simulink model "Experiment1_model"  (R2022a)
settings: Solver=FixedStepAuto  StartTime=0.0  StopTime=20  RelTol=1e-3
libraries: slpidlib x32, slctrlblks x18
(part 1 of 5)
settings Model: Creator=luca9  LastModifiedBy=luca9

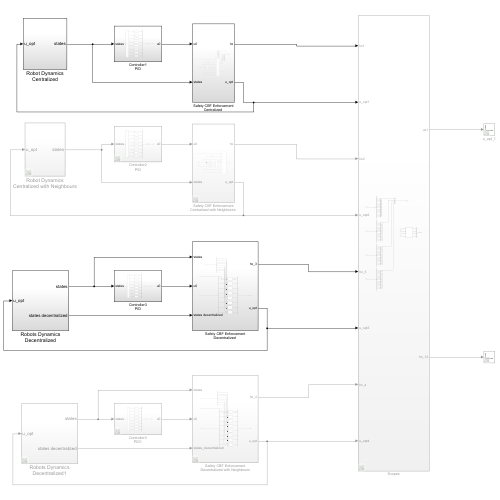
[thumbnail: Simulink's stored preview of the top-level diagram]
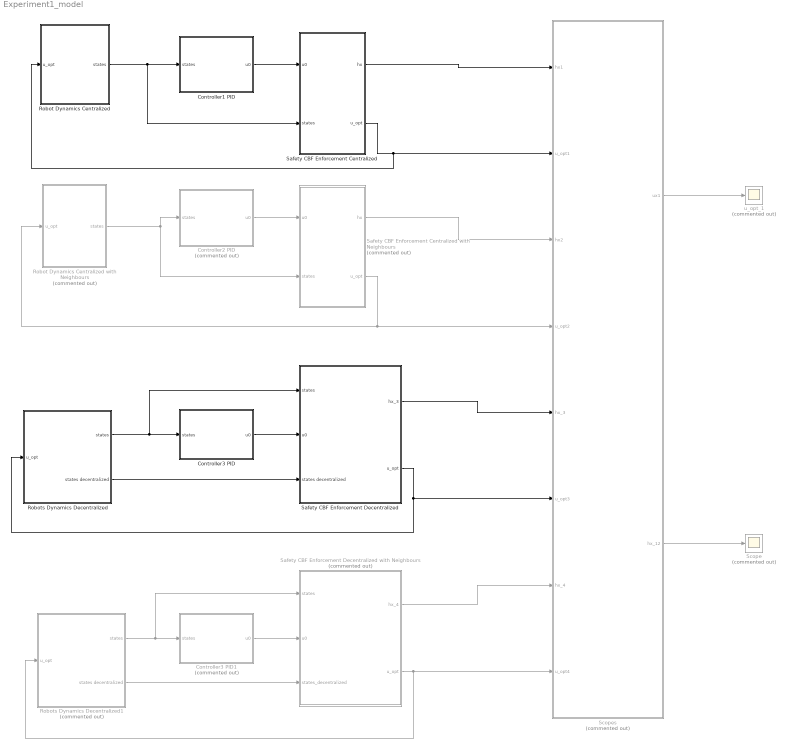
== system Experiment1_model ==
  Controller1 PID : Subsystem
  Controller2 PID : Subsystem  Commented=on
  Controller3 PID : Subsystem
  Controller3 PID1 : Subsystem  Commented=on
  "Robot Dynamics Centralized " : Subsystem
  Robot Dynamics Centralized with Neighbours : Subsystem  Commented=on
  Robots Dynamics Decentralized : Subsystem
  Robots Dynamics Decentralized1 : Subsystem  Commented=on
  "Safety CBF Enforcement Centralized " : Subsystem
  "Safety CBF Enforcement Centralized with Neighbours " : Subsystem  Commented=on
  "Safety CBF Enforcement Decentralized " : Subsystem
  "Safety CBF Enforcement Decentralized with Neighbours " : Subsystem  Commented=on
  Scope : Scope  Commented=on
  Scopes : Subsystem  Commented=on
  u_opt_1 : Scope  Commented=on
  wires:
  Controller1 PID/1(u0) -> "Safety CBF Enforcement Centralized "/1(u0)
  "Robot Dynamics Centralized "/1(states) -> Controller1 PID/1(states), "Safety CBF Enforcement Centralized "/2(states)
  Robots Dynamics Decentralized/1(states) -> "Safety CBF Enforcement Decentralized "/1(states), Controller3 PID/1(states)
  "Safety CBF Enforcement Centralized "/2(u_opt) -> "Robot Dynamics Centralized "/1(u_opt), Scopes/2(u_opt1)
  "Safety CBF Enforcement Centralized with Neighbours "/2(u_opt) -> Robot Dynamics Centralized with Neighbours/1(u_opt), Scopes/4(u_opt2)
  Robot Dynamics Centralized with Neighbours/1(states) -> Controller2 PID/1(states), "Safety CBF Enforcement Centralized with Neighbours "/2(states)
  Controller2 PID/1(u0) -> "Safety CBF Enforcement Centralized with Neighbours "/1(u0)
  "Safety CBF Enforcement Decentralized "/2(u_opt) -> Scopes/6(u_opt3), Robots Dynamics Decentralized/1(u_opt)
  Robots Dynamics Decentralized/2(states decentralized) -> "Safety CBF Enforcement Decentralized "/3(states decentralized)
  Robots Dynamics Decentralized1/1(states) -> Controller3 PID1/1(states), "Safety CBF Enforcement Decentralized with Neighbours "/1(states)
  Controller3 PID1/1(u0) -> "Safety CBF Enforcement Decentralized with Neighbours "/2(u0)
  Controller3 PID/1(u0) -> "Safety CBF Enforcement Decentralized "/2(u0)
  Robots Dynamics Decentralized1/2(states decentralized) -> "Safety CBF Enforcement Decentralized with Neighbours "/3(states_decentralized)
  "Safety CBF Enforcement Decentralized with Neighbours "/2(u_opt) -> Scopes/8(u_opt4), Robots Dynamics Decentralized1/1(u_opt)
  "Safety CBF Enforcement Centralized with Neighbours "/1(hx) -> Scopes/3(hx2)
  Scopes/1(ux1) -> u_opt_1/1
  Scopes/2(hx_12) -> Scope/1
  "Safety CBF Enforcement Centralized "/1(hx) -> Scopes/1(hx1)
  "Safety CBF Enforcement Decentralized "/1(hx_3) -> Scopes/5(hx_3)
  "Safety CBF Enforcement Decentralized with Neighbours "/1(hx_4) -> Scopes/7(hx_4)

== system Experiment1_model/Controller1 PID ==
  states : Inport
  Mux : Mux  Inputs=8
  Saturation : Saturate  UpperLimit=10  LowerLimit=-10
  Signal Routing : MATLAB Function  TreatAsAtomicUnit=on
  controller robot1 : Subsystem
  controller robot2 : Subsystem
  controller robot3 : Subsystem
  controller robot4 : Subsystem
  controller robot5 : Subsystem
  controller robot6 : Subsystem
  controller robot7 : Subsystem
  controller robot8 : Subsystem
  u0 : Outport
  wires:
  states/1 -> Signal Routing/1(states)
  Signal Routing/1(x_rob1) -> controller robot1/1(x_rob1)
  Signal Routing/2(x_rob2) -> controller robot2/1(x_rob2)
  Signal Routing/3(x_rob3) -> controller robot3/1(x_rob2)
  Signal Routing/4(x_rob4) -> controller robot4/1(x_rob2)
  Signal Routing/5(x_rob5) -> controller robot5/1(x_rob2)
  Signal Routing/6(x_rob6) -> controller robot6/1(x_rob2)
  Signal Routing/7(x_rob7) -> controller robot7/1(x_rob2)
  Signal Routing/8(x_rob8) -> controller robot8/1(x_rob2)
  controller robot1/1(u01) -> Mux/1  "u1"
  controller robot2/1(u02) -> Mux/2
  controller robot3/1(u03) -> Mux/3
  controller robot4/1(u04) -> Mux/4
  controller robot5/1(u05) -> Mux/5
  controller robot6/1(u06) -> Mux/6
  controller robot7/1(u07) -> Mux/7
  controller robot8/1(u08) -> Mux/8
  Mux/1 -> Saturation/1  "u0"
  Saturation/1 -> u0/1

== system Experiment1_model/Controller2 PID ==
  states : Inport
  Mux : Mux  Inputs=8
  Saturation : Saturate  UpperLimit=10  LowerLimit=-10
  Signal Routing : MATLAB Function  TreatAsAtomicUnit=on
  controller robot1 : Subsystem
  controller robot2 : Subsystem
  controller robot3 : Subsystem
  controller robot4 : Subsystem
  controller robot5 : Subsystem
  controller robot6 : Subsystem
  controller robot7 : Subsystem
  controller robot8 : Subsystem
  u0 : Outport
  wires:
  states/1 -> Signal Routing/1(states)
  Signal Routing/1(x_rob1) -> controller robot1/1(x_rob1)
  Signal Routing/2(x_rob2) -> controller robot2/1(x_rob2)
  Signal Routing/3(x_rob3) -> controller robot3/1(x_rob2)
  Signal Routing/4(x_rob4) -> controller robot4/1(x_rob2)
  Signal Routing/5(x_rob5) -> controller robot5/1(x_rob2)
  Signal Routing/6(x_rob6) -> controller robot6/1(x_rob2)
  Signal Routing/7(x_rob7) -> controller robot7/1(x_rob2)
  Signal Routing/8(x_rob8) -> controller robot8/1(x_rob2)
  controller robot1/1(u01) -> Mux/1  "u1"
  controller robot2/1(u02) -> Mux/2
  controller robot3/1(u03) -> Mux/3
  controller robot4/1(u04) -> Mux/4
  controller robot5/1(u05) -> Mux/5
  controller robot6/1(u06) -> Mux/6
  controller robot7/1(u07) -> Mux/7
  controller robot8/1(u08) -> Mux/8
  Mux/1 -> Saturation/1  "u0"
  Saturation/1 -> u0/1

== system Experiment1_model/Controller3 PID ==
  states : Inport
  Mux : Mux  Inputs=8
  Saturation : Saturate  UpperLimit=10  LowerLimit=-10
  Signal Routing : MATLAB Function  TreatAsAtomicUnit=on
  controller robot1 : Subsystem
  controller robot2 : Subsystem
  controller robot3 : Subsystem
  controller robot4 : Subsystem
  controller robot5 : Subsystem
  controller robot6 : Subsystem
  controller robot7 : Subsystem
  controller robot8 : Subsystem
  u0 : Outport
  wires:
  states/1 -> Signal Routing/1(states)
  Signal Routing/1(x_rob1) -> controller robot1/1(x_rob1)
  Signal Routing/2(x_rob2) -> controller robot2/1(x_rob2)
  Signal Routing/3(x_rob3) -> controller robot3/1(x_rob2)
  Signal Routing/4(x_rob4) -> controller robot4/1(x_rob2)
  Signal Routing/5(x_rob5) -> controller robot5/1(x_rob2)
  Signal Routing/6(x_rob6) -> controller robot6/1(x_rob2)
  Signal Routing/7(x_rob7) -> controller robot7/1(x_rob2)
  Signal Routing/8(x_rob8) -> controller robot8/1(x_rob2)
  controller robot1/1(u01) -> Mux/1  "u1"
  controller robot2/1(u02) -> Mux/2
  controller robot3/1(u03) -> Mux/3
  controller robot4/1(u04) -> Mux/4
  controller robot5/1(u05) -> Mux/5
  controller robot6/1(u06) -> Mux/6
  controller robot7/1(u07) -> Mux/7
  controller robot8/1(u08) -> Mux/8
  Mux/1 -> Saturation/1  "u0"
  Saturation/1 -> u0/1

== system Experiment1_model/Controller3 PID1 ==
  states : Inport
  Mux : Mux  Inputs=8
  Saturation : Saturate  UpperLimit=10  LowerLimit=-10
  Signal Routing : MATLAB Function  TreatAsAtomicUnit=on
  controller robot1 : Subsystem
  controller robot2 : Subsystem
  controller robot3 : Subsystem
  controller robot4 : Subsystem
  controller robot5 : Subsystem
  controller robot6 : Subsystem
  controller robot7 : Subsystem
  controller robot8 : Subsystem
  u0 : Outport
  wires:
  states/1 -> Signal Routing/1(states)
  Signal Routing/1(x_rob1) -> controller robot1/1(x_rob1)
  Signal Routing/2(x_rob2) -> controller robot2/1(x_rob2)
  Signal Routing/3(x_rob3) -> controller robot3/1(x_rob2)
  Signal Routing/4(x_rob4) -> controller robot4/1(x_rob2)
  Signal Routing/5(x_rob5) -> controller robot5/1(x_rob2)
  Signal Routing/6(x_rob6) -> controller robot6/1(x_rob2)
  Signal Routing/7(x_rob7) -> controller robot7/1(x_rob2)
  Signal Routing/8(x_rob8) -> controller robot8/1(x_rob2)
  controller robot1/1(u01) -> Mux/1  "u1"
  controller robot2/1(u02) -> Mux/2
  controller robot3/1(u03) -> Mux/3
  controller robot4/1(u04) -> Mux/4
  controller robot5/1(u05) -> Mux/5
  controller robot6/1(u06) -> Mux/6
  controller robot7/1(u07) -> Mux/7
  controller robot8/1(u08) -> Mux/8
  Mux/1 -> Saturation/1  "u0"
  Saturation/1 -> u0/1

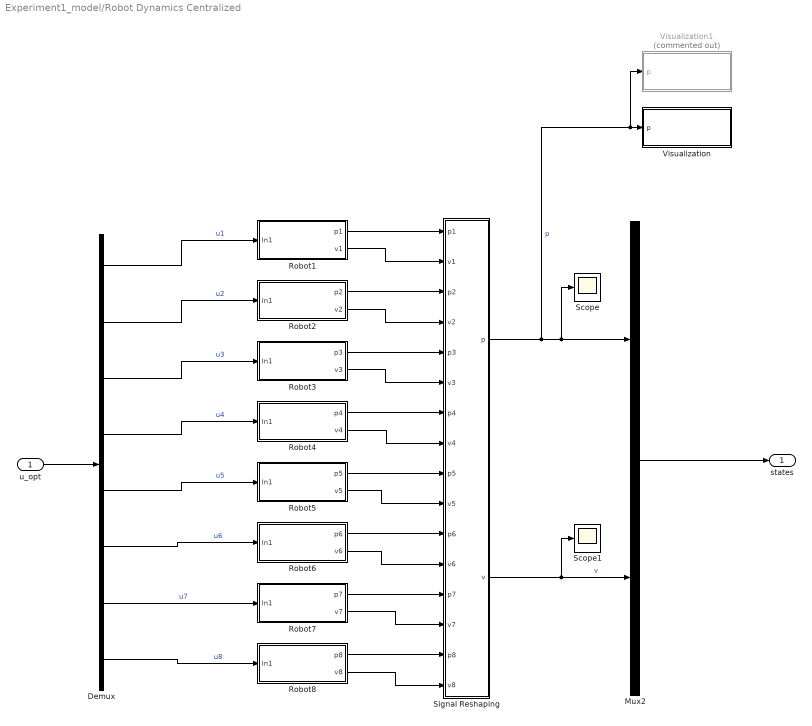
== system Experiment1_model/Robot Dynamics Centralized  ==
  u_opt : Inport
  Demux : Demux  Outputs=8
  Mux2 : Mux  Inputs=2
  Robot1 : Subsystem
  Robot2 : Subsystem
  Robot3 : Subsystem
  Robot4 : Subsystem
  Robot5 : Subsystem
  Robot6 : Subsystem
  Robot7 : Subsystem
  Robot8 : Subsystem
  Scope : Scope
  Scope1 : Scope
  Signal Reshaping : MATLAB Function  TreatAsAtomicUnit=on
  Visualization : Subsystem
  Visualization1 : Subsystem  Commented=on
  states : Outport
  wires:
  u_opt/1 -> Demux/1
  Demux/1 -> Robot1/1(In1)  "u1"
  Demux/2 -> Robot2/1(In1)  "u2"
  Demux/3 -> Robot3/1(In1)  "u3"
  Demux/4 -> Robot4/1(In1)  "u4"
  Demux/5 -> Robot5/1(In1)  "u5"
  Demux/6 -> Robot6/1(In1)  "u6"
  Demux/7 -> Robot7/1(In1)  "u7"
  Demux/8 -> Robot8/1(In1)  "u8"
  Mux2/1 -> states/1
  Signal Reshaping/2(v) -> Scope1/1, Mux2/2  "v"
  Signal Reshaping/1(p) -> Visualization1/1(p), Visualization/1(p), Scope/1, Mux2/1  "p"
  Robot1/1(p1) -> Signal Reshaping/1(p1)
  Robot1/2(v1) -> Signal Reshaping/2(v1)
  Robot2/1(p2) -> Signal Reshaping/3(p2)
  Robot2/2(v2) -> Signal Reshaping/4(v2)
  Robot3/1(p3) -> Signal Reshaping/5(p3)
  Robot3/2(v3) -> Signal Reshaping/6(v3)
  Robot4/1(p4) -> Signal Reshaping/7(p4)
  Robot4/2(v4) -> Signal Reshaping/8(v4)
  Robot5/1(p5) -> Signal Reshaping/9(p5)
  Robot5/2(v5) -> Signal Reshaping/10(v5)
  Robot6/1(p6) -> Signal Reshaping/11(p6)
  Robot6/2(v6) -> Signal Reshaping/12(v6)
  Robot7/1(p7) -> Signal Reshaping/13(p7)
  Robot7/2(v7) -> Signal Reshaping/14(v7)
  Robot8/1(p8) -> Signal Reshaping/15(p8)
  Robot8/2(v8) -> Signal Reshaping/16(v8)

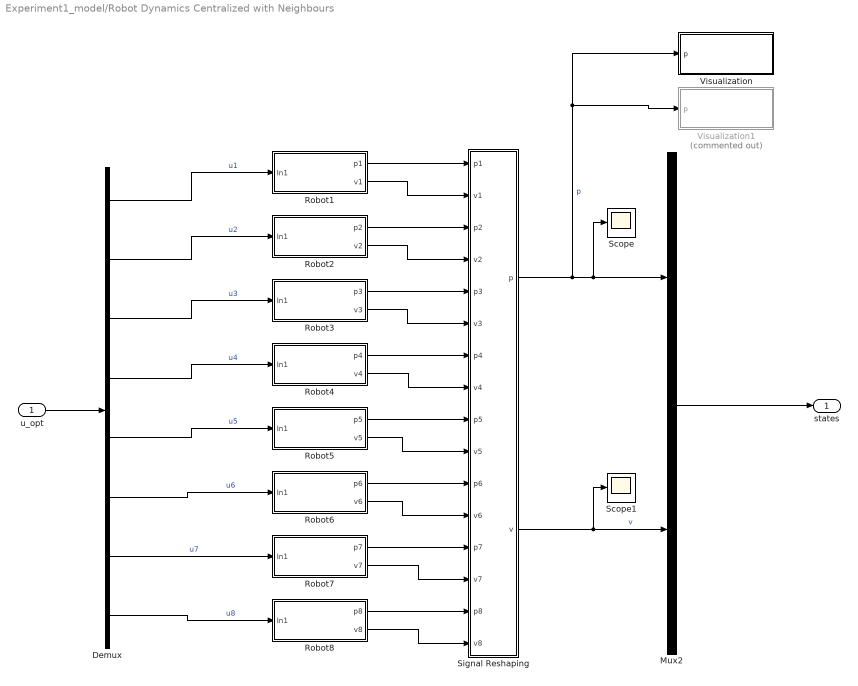
== system Experiment1_model/Robot Dynamics Centralized with Neighbours ==
  u_opt : Inport
  Demux : Demux  Outputs=8
  Mux2 : Mux  Inputs=2
  Robot1 : Subsystem
  Robot2 : Subsystem
  Robot3 : Subsystem
  Robot4 : Subsystem
  Robot5 : Subsystem
  Robot6 : Subsystem
  Robot7 : Subsystem
  Robot8 : Subsystem
  Scope : Scope
  Scope1 : Scope
  Signal Reshaping : MATLAB Function  TreatAsAtomicUnit=on
  Visualization : Subsystem
  Visualization1 : Subsystem  Commented=on
  states : Outport
  wires:
  u_opt/1 -> Demux/1
  Demux/1 -> Robot1/1(In1)  "u1"
  Demux/2 -> Robot2/1(In1)  "u2"
  Demux/3 -> Robot3/1(In1)  "u3"
  Demux/4 -> Robot4/1(In1)  "u4"
  Demux/5 -> Robot5/1(In1)  "u5"
  Demux/6 -> Robot6/1(In1)  "u6"
  Demux/7 -> Robot7/1(In1)  "u7"
  Demux/8 -> Robot8/1(In1)  "u8"
  Mux2/1 -> states/1
  Signal Reshaping/2(v) -> Scope1/1, Mux2/2  "v"
  Signal Reshaping/1(p) -> Visualization1/1(p), Visualization/1(p), Scope/1, Mux2/1  "p"
  Robot1/1(p1) -> Signal Reshaping/1(p1)
  Robot1/2(v1) -> Signal Reshaping/2(v1)
  Robot2/1(p2) -> Signal Reshaping/3(p2)
  Robot2/2(v2) -> Signal Reshaping/4(v2)
  Robot3/1(p3) -> Signal Reshaping/5(p3)
  Robot3/2(v3) -> Signal Reshaping/6(v3)
  Robot4/1(p4) -> Signal Reshaping/7(p4)
  Robot4/2(v4) -> Signal Reshaping/8(v4)
  Robot5/1(p5) -> Signal Reshaping/9(p5)
  Robot5/2(v5) -> Signal Reshaping/10(v5)
  Robot6/1(p6) -> Signal Reshaping/11(p6)
  Robot6/2(v6) -> Signal Reshaping/12(v6)
  Robot7/1(p7) -> Signal Reshaping/13(p7)
  Robot7/2(v7) -> Signal Reshaping/14(v7)
  Robot8/1(p8) -> Signal Reshaping/15(p8)
  Robot8/2(v8) -> Signal Reshaping/16(v8)

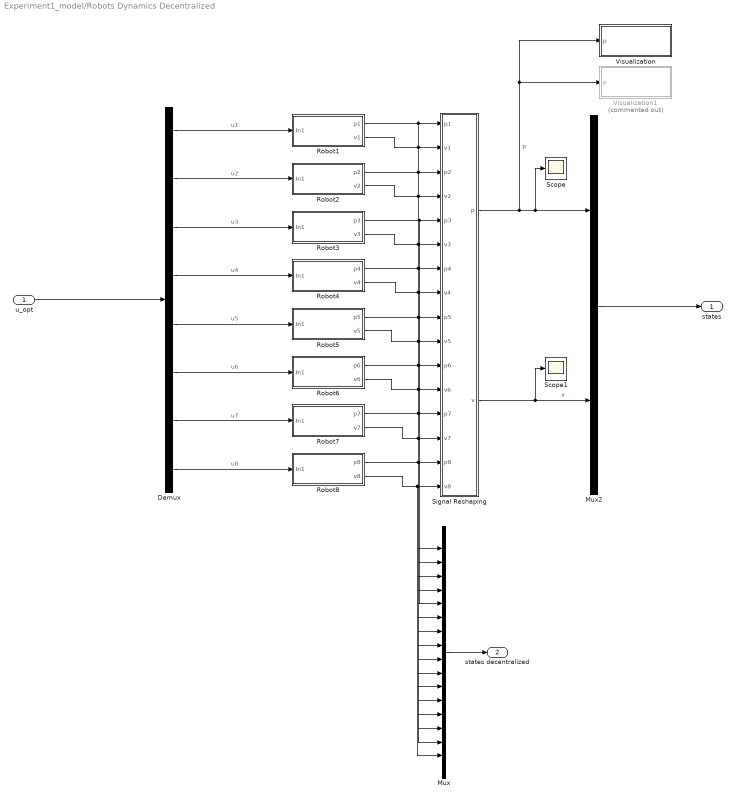
== system Experiment1_model/Robots Dynamics Decentralized ==
  u_opt : Inport
  Demux : Demux  Outputs=8
  Mux : Mux  Inputs=16
  Mux2 : Mux  Inputs=2
  Robot1 : Subsystem
  Robot2 : Subsystem
  Robot3 : Subsystem
  Robot4 : Subsystem
  Robot5 : Subsystem
  Robot6 : Subsystem
  Robot7 : Subsystem
  Robot8 : Subsystem
  Scope : Scope
  Scope1 : Scope
  Signal Reshaping : MATLAB Function  TreatAsAtomicUnit=on
  Visualization : Subsystem
  Visualization1 : Subsystem  Commented=on
  states : Outport
  states decentralized : Outport  Port=2
  wires:
  Demux/1 -> Robot1/1(In1)  "u1"
  Demux/2 -> Robot2/1(In1)  "u2"
  Demux/3 -> Robot3/1(In1)  "u3"
  Demux/4 -> Robot4/1(In1)  "u4"
  Demux/5 -> Robot5/1(In1)  "u5"
  Demux/6 -> Robot6/1(In1)  "u6"
  Demux/7 -> Robot7/1(In1)  "u7"
  Demux/8 -> Robot8/1(In1)  "u8"
  Mux2/1 -> states/1
  Signal Reshaping/2(v) -> Scope1/1, Mux2/2  "v"
  Signal Reshaping/1(p) -> Visualization1/1(p), Visualization/1(p), Scope/1, Mux2/1  "p"
  Robot1/1(p1) -> Signal Reshaping/1(p1), Mux/1
  Robot1/2(v1) -> Signal Reshaping/2(v1), Mux/2
  Robot2/1(p2) -> Signal Reshaping/3(p2), Mux/3
  Robot2/2(v2) -> Signal Reshaping/4(v2), Mux/4
  Robot3/1(p3) -> Signal Reshaping/5(p3), Mux/5
  Robot3/2(v3) -> Signal Reshaping/6(v3), Mux/6
  Robot4/1(p4) -> Signal Reshaping/7(p4), Mux/7
  Robot4/2(v4) -> Signal Reshaping/8(v4), Mux/8
  Robot5/1(p5) -> Signal Reshaping/9(p5), Mux/9
  Robot5/2(v5) -> Signal Reshaping/10(v5), Mux/10
  Robot6/1(p6) -> Signal Reshaping/11(p6), Mux/11
  Robot6/2(v6) -> Signal Reshaping/12(v6), Mux/12
  Robot7/1(p7) -> Signal Reshaping/13(p7), Mux/13
  Robot7/2(v7) -> Signal Reshaping/14(v7), Mux/14
  Robot8/1(p8) -> Signal Reshaping/15(p8), Mux/15
  Robot8/2(v8) -> Signal Reshaping/16(v8), Mux/16
  Mux/1 -> states decentralized/1
  u_opt/1 -> Demux/1

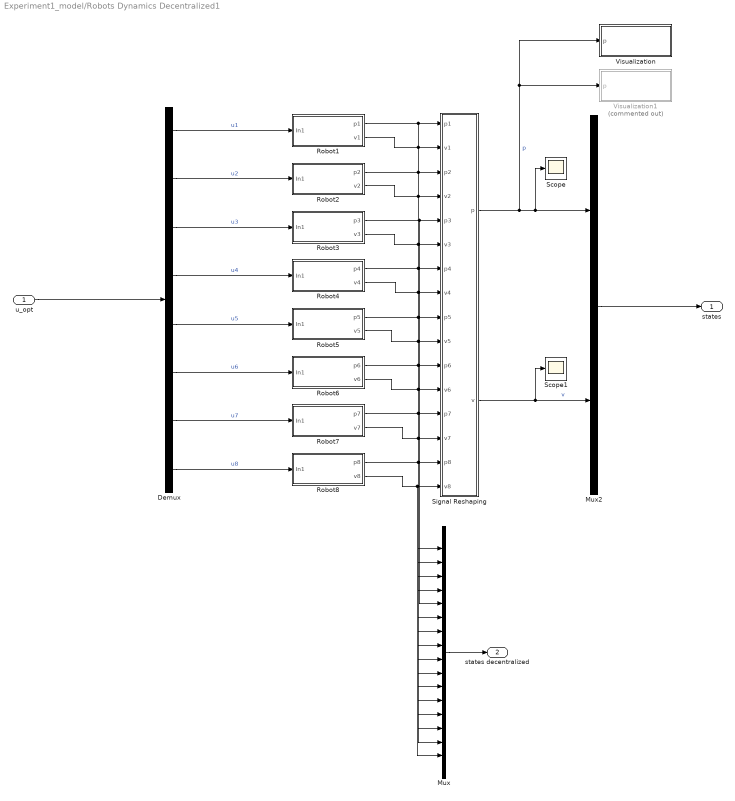
== system Experiment1_model/Robots Dynamics Decentralized1 ==
  u_opt : Inport
  Demux : Demux  Outputs=8
  Mux : Mux  Inputs=16
  Mux2 : Mux  Inputs=2
  Robot1 : Subsystem
  Robot2 : Subsystem
  Robot3 : Subsystem
  Robot4 : Subsystem
  Robot5 : Subsystem
  Robot6 : Subsystem
  Robot7 : Subsystem
  Robot8 : Subsystem
  Scope : Scope
  Scope1 : Scope
  Signal Reshaping : MATLAB Function  TreatAsAtomicUnit=on
  Visualization : Subsystem
  Visualization1 : Subsystem  Commented=on
  states : Outport
  states decentralized : Outport  Port=2
  wires:
  Demux/1 -> Robot1/1(In1)  "u1"
  Demux/2 -> Robot2/1(In1)  "u2"
  Demux/3 -> Robot3/1(In1)  "u3"
  Demux/4 -> Robot4/1(In1)  "u4"
  Demux/5 -> Robot5/1(In1)  "u5"
  Demux/6 -> Robot6/1(In1)  "u6"
  Demux/7 -> Robot7/1(In1)  "u7"
  Demux/8 -> Robot8/1(In1)  "u8"
  Mux2/1 -> states/1
  Signal Reshaping/2(v) -> Scope1/1, Mux2/2  "v"
  Signal Reshaping/1(p) -> Visualization1/1(p), Visualization/1(p), Scope/1, Mux2/1  "p"
  Robot1/1(p1) -> Signal Reshaping/1(p1), Mux/1
  Robot1/2(v1) -> Signal Reshaping/2(v1), Mux/2
  Robot2/1(p2) -> Signal Reshaping/3(p2), Mux/3
  Robot2/2(v2) -> Signal Reshaping/4(v2), Mux/4
  Robot3/1(p3) -> Signal Reshaping/5(p3), Mux/5
  Robot3/2(v3) -> Signal Reshaping/6(v3), Mux/6
  Robot4/1(p4) -> Signal Reshaping/7(p4), Mux/7
  Robot4/2(v4) -> Signal Reshaping/8(v4), Mux/8
  Robot5/1(p5) -> Signal Reshaping/9(p5), Mux/9
  Robot5/2(v5) -> Signal Reshaping/10(v5), Mux/10
  Robot6/1(p6) -> Signal Reshaping/11(p6), Mux/11
  Robot6/2(v6) -> Signal Reshaping/12(v6), Mux/12
  Robot7/1(p7) -> Signal Reshaping/13(p7), Mux/13
  Robot7/2(v7) -> Signal Reshaping/14(v7), Mux/14
  Robot8/1(p8) -> Signal Reshaping/15(p8), Mux/15
  Robot8/2(v8) -> Signal Reshaping/16(v8), Mux/16
  Mux/1 -> states decentralized/1
  u_opt/1 -> Demux/1

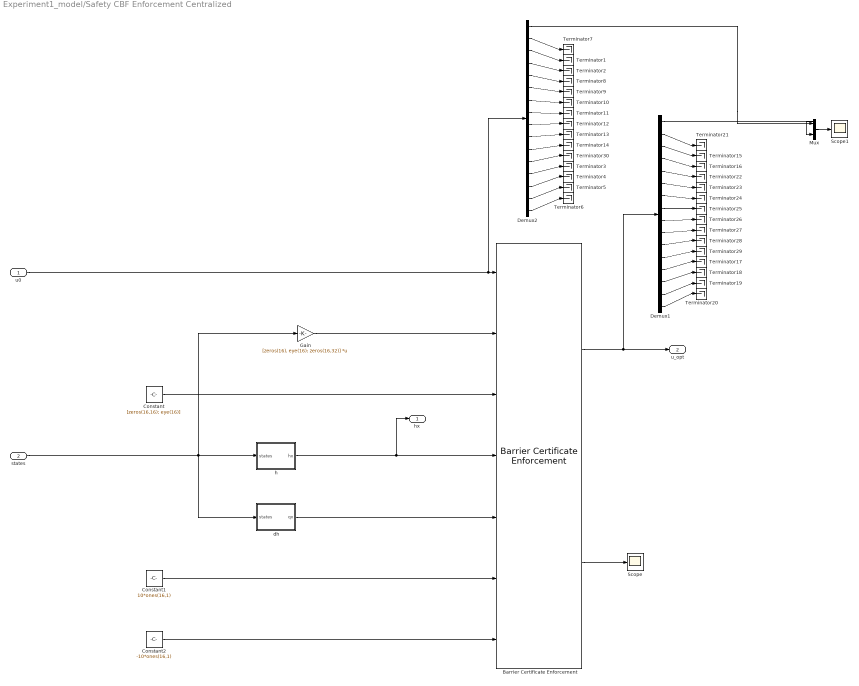
== system Experiment1_model/Safety CBF Enforcement Centralized  ==
  u0 : Inport
  states : Inport  Port=2
  Barrier Certificate Enforcement : slctrlblks/Barrier Certificate Enforcement  nx=32  nu=16  nc=28  gamma=0.005  beta=3  external_umax=on  external_umin=on  Ts=0.1  maxiter=200  tol=1e-6  output_exitflag=on
      settings: SourceProductBaseCode=SD
  Constant : Constant  Value=[zeros(16,16); eye(16)]
  Constant1 : Constant  Value=10*ones(16,1)
  Constant2 : Constant  Value=-10*ones(16,1)
  Demux1 : Demux  Outputs=16
  Demux2 : Demux  Outputs=16
  Gain : Gain  Gain=[zeros(16), eye(16); zeros(16,32)]  Multiplication=Matrix(K*u)
  Mux : Mux  Inputs=2
  Scope : Scope
  Scope1 : Scope
  Terminator{1..30} (30 alike) : Terminator
  dh : MATLAB Function  TreatAsAtomicUnit=on
  h : MATLAB Function  TreatAsAtomicUnit=on
  hx : Outport
  u_opt : Outport  Port=2
  wires:
  Barrier Certificate Enforcement/1 -> Demux1/1, u_opt/1
  u0/1 -> Demux2/1, Barrier Certificate Enforcement/1
  states/1 -> Gain/1, h/1(states), dh/1(states)
  Constant/1 -> Barrier Certificate Enforcement/3
  Gain/1 -> Barrier Certificate Enforcement/2
  Constant1/1 -> Barrier Certificate Enforcement/6
  Constant2/1 -> Barrier Certificate Enforcement/7
  h/1(hx) -> hx/1, Barrier Certificate Enforcement/4
  dh/1(qx) -> Barrier Certificate Enforcement/5
  Barrier Certificate Enforcement/2 -> Scope/1
  Mux/1 -> Scope1/1
  Demux1/5 -> Terminator22/1
  Demux1/2 -> Terminator21/1
  Demux1/7 -> Terminator24/1
  Demux1/10 -> Terminator27/1
  Demux1/13 -> Terminator17/1
  Demux1/16 -> Terminator20/1
  Demux1/9 -> Terminator26/1
  Demux1/12 -> Terminator29/1
  Demux1/8 -> Terminator25/1
  Demux1/3 -> Terminator15/1
  Demux1/14 -> Terminator18/1
  Demux1/4 -> Terminator16/1
  Demux1/11 -> Terminator28/1
  Demux1/6 -> Terminator23/1
  Demux1/15 -> Terminator19/1
  Demux1/1 -> Mux/2
  Demux2/5 -> Terminator8/1
  Demux2/2 -> Terminator7/1
  Demux2/7 -> Terminator10/1
  Demux2/10 -> Terminator13/1
  Demux2/13 -> Terminator3/1
  Demux2/16 -> Terminator6/1
  Demux2/9 -> Terminator12/1
  Demux2/12 -> Terminator30/1
  Demux2/8 -> Terminator11/1
  Demux2/3 -> Terminator1/1
  Demux2/14 -> Terminator4/1
  Demux2/4 -> Terminator2/1
  Demux2/11 -> Terminator14/1
  Demux2/6 -> Terminator9/1
  Demux2/15 -> Terminator5/1
  Demux2/1 -> Mux/1

== system Experiment1_model/Safety CBF Enforcement Centralized with Neighbours  ==
  u0 : Inport
  states : Inport  Port=2
  Barrier Certificate Enforcement : slctrlblks/Barrier Certificate Enforcement  nx=32  nu=16  nc=28  gamma=0.005  beta=3  external_umax=on  external_umin=on  Ts=0.1  maxiter=200  tol=1e-6  output_exitflag=off
      settings: SourceProductBaseCode=SD
  Constant : Constant  Value=[zeros(16,16); eye(16)]
  Constant1 : Constant  Value=10*ones(16,1)
  Constant2 : Constant  Value=-10*ones(16,1)
  DeltaP : MATLAB Function  TreatAsAtomicUnit=on
  Gain : Gain  Gain=[zeros(16), eye(16); zeros(16,32)]  Multiplication=Matrix(K*u)
  MATLAB Function1 : MATLAB Function  TreatAsAtomicUnit=on
  dh : MATLAB Function  TreatAsAtomicUnit=on
  h : MATLAB Function  TreatAsAtomicUnit=on
  hx : Outport
  u_opt : Outport  Port=2
  wires:
  Barrier Certificate Enforcement/1 -> u_opt/1
  u0/1 -> Barrier Certificate Enforcement/1
  states/1 -> Gain/1, h/1(states), dh/1(states), DeltaP/1(states)
  Constant/1 -> Barrier Certificate Enforcement/3
  Gain/1 -> Barrier Certificate Enforcement/2
  Constant1/1 -> Barrier Certificate Enforcement/6
  Constant2/1 -> Barrier Certificate Enforcement/7
  MATLAB Function1/1(hx) -> hx/1, Barrier Certificate Enforcement/4
  MATLAB Function1/2(qx) -> Barrier Certificate Enforcement/5
  h/1(hx) -> MATLAB Function1/1("hx ")
  dh/1(qx) -> MATLAB Function1/2("qx ")
  DeltaP/1(deltaP) -> MATLAB Function1/3(deltaP)

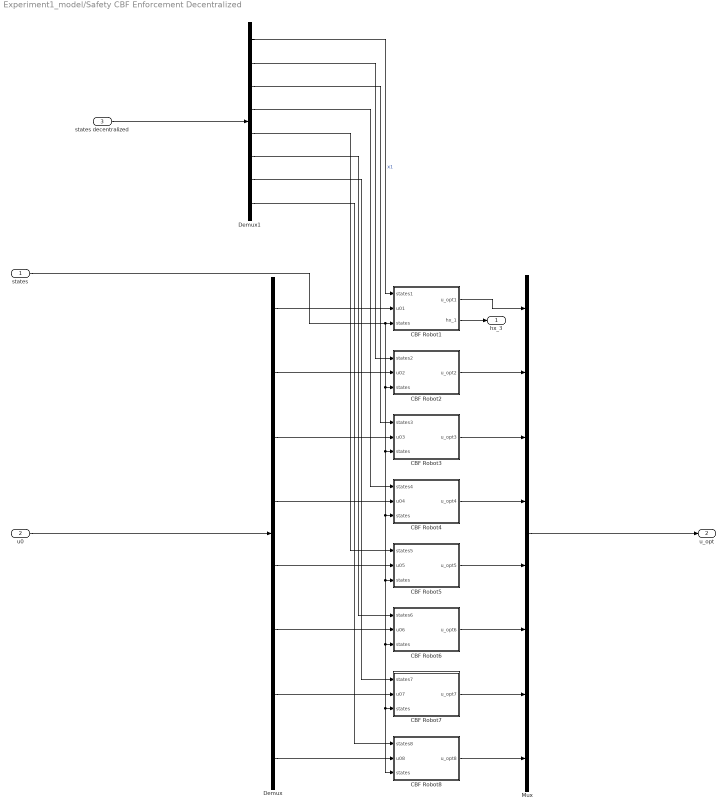
== system Experiment1_model/Safety CBF Enforcement Decentralized  ==
  states : Inport
  u0 : Inport  Port=2
  states decentralized : Inport  Port=3
  CBF Robot1 : Subsystem
  CBF Robot2 : Subsystem
  CBF Robot3 : Subsystem
  CBF Robot4 : Subsystem
  CBF Robot5 : Subsystem
  CBF Robot6 : Subsystem
  CBF Robot7 : Subsystem
  CBF Robot8 : Subsystem
  Demux : Demux  Outputs=8
  Demux1 : Demux  Outputs=8
  Mux : Mux  Inputs=8
  hx_3 : Outport
  u_opt : Outport  Port=2
  wires:
  states/1 -> CBF Robot8/3(states), CBF Robot7/3(states), CBF Robot6/3(states), CBF Robot5/3(states), CBF Robot4/3(states), CBF Robot3/3(states), CBF Robot2/3(states), CBF Robot1/3(states)
  Demux1/1 -> CBF Robot1/1(states1)  "x1"
  CBF Robot1/1(u_opt1) -> Mux/1
  Demux/1 -> CBF Robot1/2(u01)
  u0/1 -> Demux/1
  Mux/1 -> u_opt/1
  states decentralized/1 -> Demux1/1
  Demux/8 -> CBF Robot8/2(u08)
  Demux/7 -> CBF Robot7/2(u07)
  Demux/6 -> CBF Robot6/2(u06)
  Demux/5 -> CBF Robot5/2(u05)
  Demux/4 -> CBF Robot4/2(u04)
  Demux/3 -> CBF Robot3/2(u03)
  Demux/2 -> CBF Robot2/2(u02)
  CBF Robot8/1(u_opt8) -> Mux/8
  CBF Robot7/1(u_opt7) -> Mux/7
  CBF Robot2/1(u_opt2) -> Mux/2
  CBF Robot3/1(u_opt3) -> Mux/3
  CBF Robot4/1(u_opt4) -> Mux/4
  CBF Robot5/1(u_opt5) -> Mux/5
  CBF Robot6/1(u_opt6) -> Mux/6
  Demux1/2 -> CBF Robot2/1(states2)
  Demux1/3 -> CBF Robot3/1(states3)
  Demux1/4 -> CBF Robot4/1(states4)
  Demux1/5 -> CBF Robot5/1(states5)
  Demux1/6 -> CBF Robot6/1(states6)
  Demux1/7 -> CBF Robot7/1(states7)
  Demux1/8 -> CBF Robot8/1(states8)
  CBF Robot1/2(hx_1) -> hx_3/1

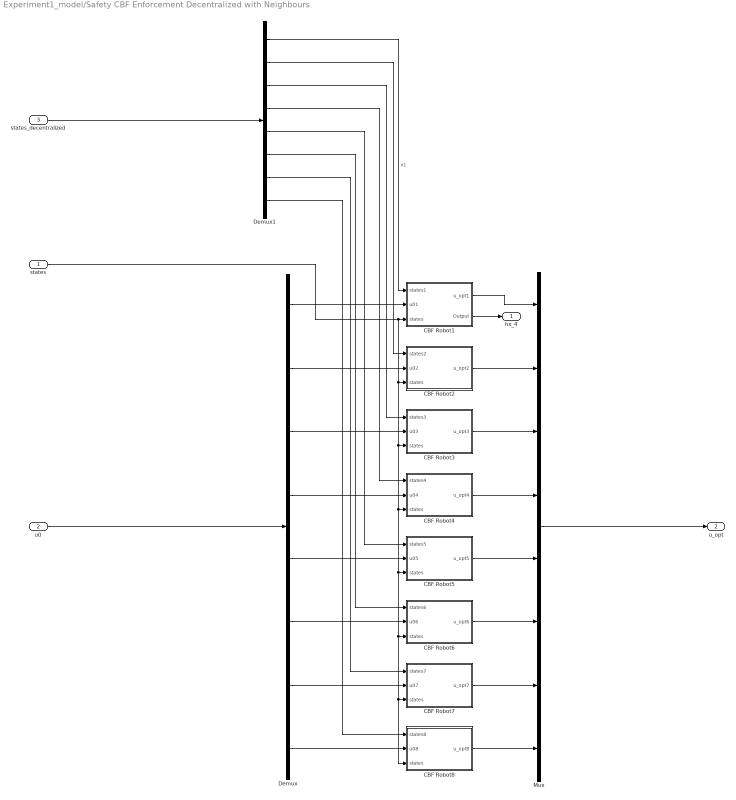
== system Experiment1_model/Safety CBF Enforcement Decentralized with Neighbours  ==
  states : Inport
  u0 : Inport  Port=2
  states_decentralized : Inport  Port=3
  CBF Robot1 : Subsystem
  CBF Robot2 : Subsystem
  CBF Robot3 : Subsystem
  CBF Robot4 : Subsystem
  CBF Robot5 : Subsystem
  CBF Robot6 : Subsystem
  CBF Robot7 : Subsystem
  CBF Robot8 : Subsystem
  Demux : Demux  Outputs=8
  Demux1 : Demux  Outputs=8
  Mux : Mux  Inputs=8
  hx_4 : Outport
  u_opt : Outport  Port=2
  wires:
  states/1 -> CBF Robot8/3(states), CBF Robot7/3(states), CBF Robot6/3(states), CBF Robot5/3(states), CBF Robot4/3(states), CBF Robot3/3(states), CBF Robot2/3(states), CBF Robot1/3(states)
  Demux1/1 -> CBF Robot1/1(states1)  "x1"
  CBF Robot1/1(u_opt1) -> Mux/1
  Demux/1 -> CBF Robot1/2(u01)
  u0/1 -> Demux/1
  Mux/1 -> u_opt/1
  states_decentralized/1 -> Demux1/1
  Demux/8 -> CBF Robot8/2(u08)
  Demux/7 -> CBF Robot7/2(u07)
  Demux/6 -> CBF Robot6/2(u06)
  Demux/5 -> CBF Robot5/2(u05)
  Demux/4 -> CBF Robot4/2(u04)
  Demux/3 -> CBF Robot3/2(u03)
  Demux/2 -> CBF Robot2/2(u02)
  CBF Robot8/1(u_opt8) -> Mux/8
  CBF Robot7/1(u_opt7) -> Mux/7
  CBF Robot2/1(u_opt2) -> Mux/2
  CBF Robot3/1(u_opt3) -> Mux/3
  CBF Robot4/1(u_opt4) -> Mux/4
  CBF Robot5/1(u_opt5) -> Mux/5
  CBF Robot6/1(u_opt6) -> Mux/6
  Demux1/2 -> CBF Robot2/1(states2)
  Demux1/3 -> CBF Robot3/1(states3)
  Demux1/4 -> CBF Robot4/1(states4)
  Demux1/5 -> CBF Robot5/1(states5)
  Demux1/6 -> CBF Robot6/1(states6)
  Demux1/7 -> CBF Robot7/1(states7)
  Demux1/8 -> CBF Robot8/1(states8)
  CBF Robot1/2(Output) -> hx_4/1

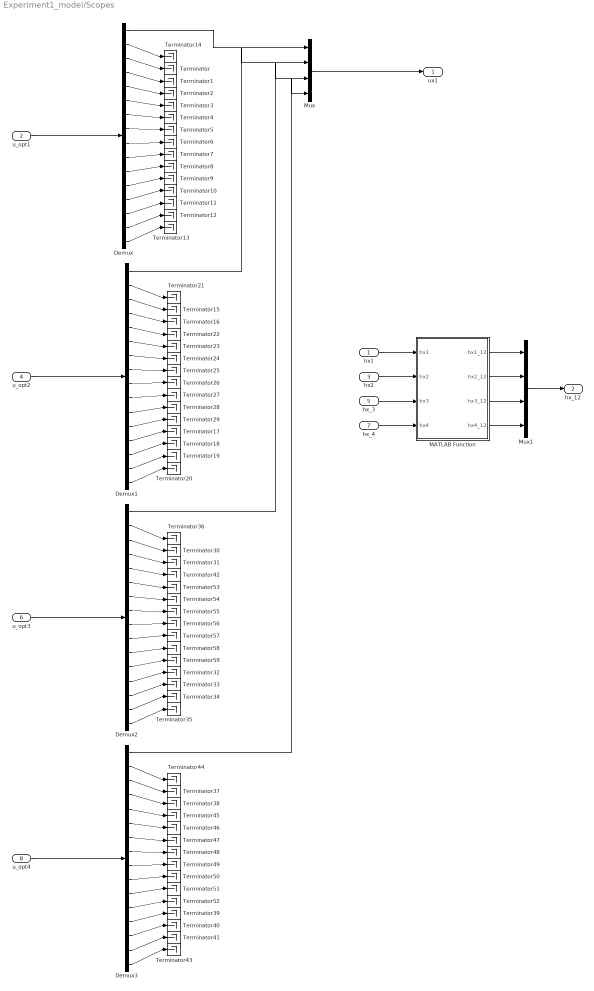
== system Experiment1_model/Scopes ==
  hx1 : Inport
  u_opt1 : Inport  Port=2
  hx2 : Inport  Port=3
  u_opt2 : Inport  Port=4
  hx_3 : Inport  Port=5
  u_opt3 : Inport  Port=6
  hx_4 : Inport  Port=7
  u_opt4 : Inport  Port=8
  Demux{,1..3} (4 alike) : Demux  Outputs=16
  MATLAB Function : MATLAB Function  TreatAsAtomicUnit=on
  Mux : Mux
  Mux1 : Mux
  Terminator{,1..59} (60 alike) : Terminator
  ux1 : Outport
  hx_12 : Outport  Port=2
  wires:
  Demux/3 -> Terminator/1
  u_opt2/1 -> Demux1/1
  Demux/8 -> Terminator5/1
  Demux/2 -> Terminator14/1
  Demux/5 -> Terminator2/1
  u_opt1/1 -> Demux/1
  Demux1/10 -> Terminator27/1
  Demux/10 -> Terminator7/1
  Demux/12 -> Terminator9/1
  Demux1/8 -> Terminator25/1
  Demux/15 -> Terminator12/1
  Demux/16 -> Terminator13/1
  Demux/9 -> Terminator6/1
  Demux/7 -> Terminator4/1
  Mux/1 -> ux1/1
  Demux/6 -> Terminator3/1
  Demux/11 -> Terminator8/1
  Demux/14 -> Terminator11/1
  Demux1/12 -> Terminator29/1
  Demux1/14 -> Terminator18/1
  Demux/13 -> Terminator10/1
  Demux/4 -> Terminator1/1
  Demux1/3 -> Terminator15/1
  Demux1/2 -> Terminator21/1
  Demux1/4 -> Terminator16/1
  Demux1/7 -> Terminator24/1
  Demux1/5 -> Terminator22/1
  Demux1/15 -> Terminator19/1
  Demux1/9 -> Terminator26/1
  Demux1/6 -> Terminator23/1
  Demux1/11 -> Terminator28/1
  Demux1/13 -> Terminator17/1
  Demux1/16 -> Terminator20/1
  hx1/1 -> MATLAB Function/1(hx1)
  hx2/1 -> MATLAB Function/2(hx2)
  Mux1/1 -> hx_12/1
  Demux2/4 -> Terminator31/1
  Demux3/13 -> Terminator39/1
  Demux2/15 -> Terminator34/1
  Demux3/6 -> Terminator46/1
  u_opt3/1 -> Demux2/1
  Demux3/3 -> Terminator37/1
  Demux2/3 -> Terminator30/1
  Demux2/13 -> Terminator32/1
  Demux3/5 -> Terminator45/1
  Demux3/11 -> Terminator51/1
  Demux3/15 -> Terminator41/1
  Demux2/11 -> Terminator58/1
  Demux3/16 -> Terminator43/1
  Demux3/9 -> Terminator49/1
  Demux2/9 -> Terminator56/1
  Demux3/12 -> Terminator52/1
  Demux2/14 -> Terminator33/1
  Demux2/5 -> Terminator42/1
  Demux3/7 -> Terminator47/1
  Demux3/4 -> Terminator38/1
  Demux3/2 -> Terminator44/1
  Demux2/6 -> Terminator53/1
  Demux3/10 -> Terminator50/1
  Demux2/7 -> Terminator54/1
  Demux2/8 -> Terminator55/1
  Demux2/10 -> Terminator57/1
  Demux2/12 -> Terminator59/1
  Demux2/16 -> Terminator35/1
  Demux2/2 -> Terminator36/1
  Demux3/14 -> Terminator40/1
  u_opt4/1 -> Demux3/1
  Demux3/8 -> Terminator48/1
  Demux/1 -> Mux/1
  Demux1/1 -> Mux/2
  hx_4/1 -> MATLAB Function/4(hx4)
  hx_3/1 -> MATLAB Function/3(hx3)
  MATLAB Function/1(hx1_12) -> Mux1/1
  MATLAB Function/2(hx2_12) -> Mux1/2
  MATLAB Function/3(hx3_12) -> Mux1/3
  MATLAB Function/4(hx4_12) -> Mux1/4
  Demux2/1 -> Mux/3
  Demux3/1 -> Mux/4

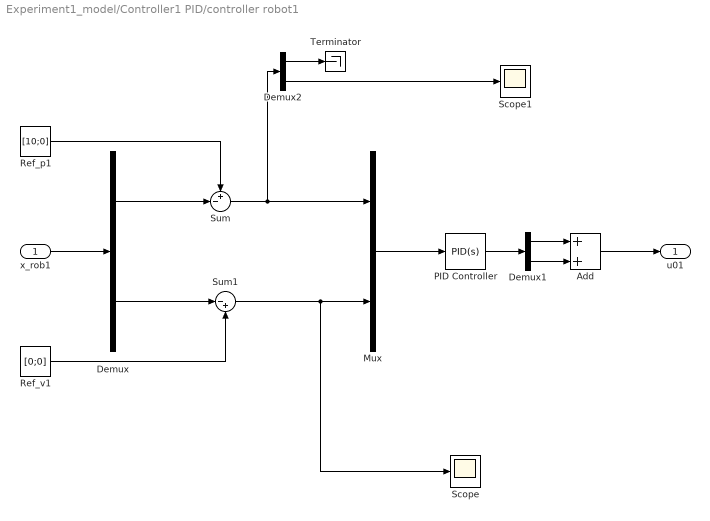
== system Experiment1_model/Controller1 PID/controller robot1 ==
  x_rob1 : Inport
  Add : Sum
  Demux : Demux  Outputs=2
  Demux1 : Demux  Outputs=2
  Demux2 : Demux  Outputs=2
  Mux : Mux  Inputs=2
  PID Controller : slpidlib/PID Controller  Controller=PID  Form=Parallel  TimeDomain=Continuous-time  UseExternalTs=off  SampleTime=-1  IntegratorMethod=Forward Euler  FilterMethod=Forward Euler  ControllerParametersSource=internal  P=5  I=0.0000001  UseKiTs=off  D=0.01  N=1  UseFilter=on  TunerSelectOption=Transfer Function Based (PID Tuner App)  InitialConditionSource=internal  InitialConditionForIntegrator=0  InitialConditionForFilter=0  DifferentiatorICPrevScaledInput=0  ExternalReset=none  TrackingMode=off  Kt=1  LimitOutput=off  SatLimitsSource=internal  UpperSaturationLimit=inf  LowerSaturationLimit=-inf  LinearizeAsGain=on  AntiWindupMode=none  Kb=1  POutMin=[]  POutMax=[]  IOutMin=[]  IOutMax=[]  DOutMin=[]  DOutMax=[]  NOutMin=[]  NOutMax=[]  SumOutMin=[]  SumOutMax=[]  SaturationOutMin=[]  SaturationOutMax=[]  PParamMin=[]  PParamMax=[]  IParamMin=[]  IParamMax=[]  DParamMin=[]  DParamMax=[]  NParamMin=[]  NParamMax=[]  KbParamMin=[]  KbParamMax=[]  KtParamMin=[]  KtParamMax=[]  KbOutMin=[]  KbOutMax=[]  KtOutMin=[]  KtOutMax=[]  IntegratorOutMin=[]  IntegratorOutMax=[]  FilterOutMin=[]  FilterOutMax=[]  SumI1OutMin=[]  SumI1OutMax=[]  SumI2OutMin=[]  SumI2OutMax=[]  SumI3OutMin=[]  SumI3OutMax=[]  SumI4OutMin=[]  SumI4OutMax=[]  SumDOutMin=[]  SumDOutMax=[]  DifferentiatorOutMin=[]  DifferentiatorOutMax=[]  FilterDiffOutCoefMin=[]  FilterDiffOutCoefMax=[]  ReciprocalOutMin=[]  ReciprocalOutMax=[]  SumDenOutMin=[]  SumDenOutMax=[]  SumNumOutMin=[]  SumNumOutMax=[]  DivideOutMin=[]  DivideOutMax=[]  UdiffTsProdOutMin=[]  UdiffTsProdOutMax=[]  NTsProdOutMin=[]  NTsProdOutMax=[]  UintegralTsProdOutMin=[]  UintegralTsProdOutMax=[]  UngainTsProdOutMin=[]  UngainTsProdOutMax=[]  IntegratorContinuousStateAttributes=''  IntegratorStateMustResolveToSignalObject=off  IntegratorRTWStateStorageClass=Auto  FilterContinuousStateAttributes=''  FilterStateMustResolveToSignalObject=off  FilterRTWStateStorageClass=Auto  ParallelPVariant=InternalParameters  IdealPVariant=Disabled  IVariant=InternalParameters  DVariant=InternalParameters  IntegratorVariant=Continuous  SatVariant=Disabled  AWVariant=Passthrough  PCopyVariant=Disabled  TRVariant=Disabled  FdbkBlocksVariant=Forward  IdealPFdbkVariant=Disabled  SatFdbkVariant=Disabled  DerivativeFilterVariant=ContFilter  NVariant=InternalParameters  NCopyVariant=Disabled  FilterICVariant=InternalICsFilter  IntegratorICVariant=InternalICs  ExternalResetVariant=Disabled  TRSumVariant=Passthrough  SumFdbkVariant=Disabled  SumVariant=Sum_PID  TsampFilterVariant=InternalTs  TsampNgainVariant=Passthrough  TsampIntegralVariant=Passthrough  ExternalSaturationOutDataTypeStr=Inherit: Same as second input  aMode=0
  Ref_p1 : Constant  Value=[10;0]  VectorParams1D=off
  Ref_v1 : Constant  Value=[0;0]  VectorParams1D=off
  Scope : Scope
  Scope1 : Scope
  Sum : Sum  Inputs=+-|
  Sum1 : Sum  Inputs=|-+
  Terminator : Terminator
  u01 : Outport
  wires:
  x_rob1/1 -> Demux/1
  Demux/1 -> Sum/2
  Ref_p1/1 -> Sum/1
  Demux/2 -> Sum1/1
  Ref_v1/1 -> Sum1/2
  Sum/1 -> Mux/1, Demux2/1
  Sum1/1 -> Mux/2, Scope/1
  Mux/1 -> PID Controller/1
  PID Controller/1 -> Demux1/1
  Demux1/2 -> Add/2
  Demux1/1 -> Add/1
  Add/1 -> u01/1
  Demux2/1 -> Terminator/1
  Demux2/2 -> Scope1/1

== system Experiment1_model/Controller1 PID/controller robot2 ==
  x_rob2 : Inport
  Add : Sum
  Demux : Demux  Outputs=2
  Demux1 : Demux  Outputs=2
  Mux : Mux  Inputs=2
  PID Controller : slpidlib/PID Controller  Controller=PID  Form=Parallel  TimeDomain=Continuous-time  UseExternalTs=off  SampleTime=-1  IntegratorMethod=Forward Euler  FilterMethod=Forward Euler  ControllerParametersSource=internal  P=5  I=0.0000001  UseKiTs=off  D=0.01  N=1  UseFilter=on  TunerSelectOption=Transfer Function Based (PID Tuner App)  InitialConditionSource=internal  InitialConditionForIntegrator=0  InitialConditionForFilter=0  DifferentiatorICPrevScaledInput=0  ExternalReset=none  TrackingMode=off  Kt=1  LimitOutput=off  SatLimitsSource=internal  UpperSaturationLimit=inf  LowerSaturationLimit=-inf  LinearizeAsGain=on  AntiWindupMode=none  Kb=1  POutMin=[]  POutMax=[]  IOutMin=[]  IOutMax=[]  DOutMin=[]  DOutMax=[]  NOutMin=[]  NOutMax=[]  SumOutMin=[]  SumOutMax=[]  SaturationOutMin=[]  SaturationOutMax=[]  PParamMin=[]  PParamMax=[]  IParamMin=[]  IParamMax=[]  DParamMin=[]  DParamMax=[]  NParamMin=[]  NParamMax=[]  KbParamMin=[]  KbParamMax=[]  KtParamMin=[]  KtParamMax=[]  KbOutMin=[]  KbOutMax=[]  KtOutMin=[]  KtOutMax=[]  IntegratorOutMin=[]  IntegratorOutMax=[]  FilterOutMin=[]  FilterOutMax=[]  SumI1OutMin=[]  SumI1OutMax=[]  SumI2OutMin=[]  SumI2OutMax=[]  SumI3OutMin=[]  SumI3OutMax=[]  SumI4OutMin=[]  SumI4OutMax=[]  SumDOutMin=[]  SumDOutMax=[]  DifferentiatorOutMin=[]  DifferentiatorOutMax=[]  FilterDiffOutCoefMin=[]  FilterDiffOutCoefMax=[]  ReciprocalOutMin=[]  ReciprocalOutMax=[]  SumDenOutMin=[]  SumDenOutMax=[]  SumNumOutMin=[]  SumNumOutMax=[]  DivideOutMin=[]  DivideOutMax=[]  UdiffTsProdOutMin=[]  UdiffTsProdOutMax=[]  NTsProdOutMin=[]  NTsProdOutMax=[]  UintegralTsProdOutMin=[]  UintegralTsProdOutMax=[]  UngainTsProdOutMin=[]  UngainTsProdOutMax=[]  IntegratorContinuousStateAttributes=''  IntegratorStateMustResolveToSignalObject=off  IntegratorRTWStateStorageClass=Auto  FilterContinuousStateAttributes=''  FilterStateMustResolveToSignalObject=off  FilterRTWStateStorageClass=Auto  ParallelPVariant=InternalParameters  IdealPVariant=Disabled  IVariant=InternalParameters  DVariant=InternalParameters  IntegratorVariant=Continuous  SatVariant=Disabled  AWVariant=Passthrough  PCopyVariant=Disabled  TRVariant=Disabled  FdbkBlocksVariant=Forward  IdealPFdbkVariant=Disabled  SatFdbkVariant=Disabled  DerivativeFilterVariant=ContFilter  NVariant=InternalParameters  NCopyVariant=Disabled  FilterICVariant=InternalICsFilter  IntegratorICVariant=InternalICs  ExternalResetVariant=Disabled  TRSumVariant=Passthrough  SumFdbkVariant=Disabled  SumVariant=Sum_PID  TsampFilterVariant=InternalTs  TsampNgainVariant=Passthrough  TsampIntegralVariant=Passthrough  ExternalSaturationOutDataTypeStr=Inherit: Same as second input  aMode=0
  Ref_p1 : Constant  Value=[8;8]  VectorParams1D=off
  Ref_v1 : Constant  Value=[0;0]  VectorParams1D=off
  Scope : Scope
  Sum : Sum  Inputs=+-|
  Sum1 : Sum  Inputs=|-+
  u02 : Outport
  wires:
  x_rob2/1 -> Demux/1
  Demux/1 -> Sum/2
  Ref_p1/1 -> Sum/1
  Demux/2 -> Sum1/1
  Ref_v1/1 -> Sum1/2
  Add/1 -> u02/1
  Demux1/2 -> Add/2
  Mux/1 -> PID Controller/1
  Sum/1 -> Scope/1, Mux/1
  Sum1/1 -> Mux/2
  PID Controller/1 -> Demux1/1
  Demux1/1 -> Add/1

== system Experiment1_model/Controller1 PID/controller robot3 ==
  x_rob2 : Inport
  Add : Sum
  Demux : Demux  Outputs=2
  Demux1 : Demux  Outputs=2
  Mux : Mux  Inputs=2
  PID Controller : slpidlib/PID Controller  Controller=PID  Form=Parallel  TimeDomain=Continuous-time  UseExternalTs=off  SampleTime=-1  IntegratorMethod=Forward Euler  FilterMethod=Forward Euler  ControllerParametersSource=internal  P=5  I=0.0000001  UseKiTs=off  D=0.01  N=1  UseFilter=on  TunerSelectOption=Transfer Function Based (PID Tuner App)  InitialConditionSource=internal  InitialConditionForIntegrator=0  InitialConditionForFilter=0  DifferentiatorICPrevScaledInput=0  ExternalReset=none  TrackingMode=off  Kt=1  LimitOutput=off  SatLimitsSource=internal  UpperSaturationLimit=inf  LowerSaturationLimit=-inf  LinearizeAsGain=on  AntiWindupMode=none  Kb=1  POutMin=[]  POutMax=[]  IOutMin=[]  IOutMax=[]  DOutMin=[]  DOutMax=[]  NOutMin=[]  NOutMax=[]  SumOutMin=[]  SumOutMax=[]  SaturationOutMin=[]  SaturationOutMax=[]  PParamMin=[]  PParamMax=[]  IParamMin=[]  IParamMax=[]  DParamMin=[]  DParamMax=[]  NParamMin=[]  NParamMax=[]  KbParamMin=[]  KbParamMax=[]  KtParamMin=[]  KtParamMax=[]  KbOutMin=[]  KbOutMax=[]  KtOutMin=[]  KtOutMax=[]  IntegratorOutMin=[]  IntegratorOutMax=[]  FilterOutMin=[]  FilterOutMax=[]  SumI1OutMin=[]  SumI1OutMax=[]  SumI2OutMin=[]  SumI2OutMax=[]  SumI3OutMin=[]  SumI3OutMax=[]  SumI4OutMin=[]  SumI4OutMax=[]  SumDOutMin=[]  SumDOutMax=[]  DifferentiatorOutMin=[]  DifferentiatorOutMax=[]  FilterDiffOutCoefMin=[]  FilterDiffOutCoefMax=[]  ReciprocalOutMin=[]  ReciprocalOutMax=[]  SumDenOutMin=[]  SumDenOutMax=[]  SumNumOutMin=[]  SumNumOutMax=[]  DivideOutMin=[]  DivideOutMax=[]  UdiffTsProdOutMin=[]  UdiffTsProdOutMax=[]  NTsProdOutMin=[]  NTsProdOutMax=[]  UintegralTsProdOutMin=[]  UintegralTsProdOutMax=[]  UngainTsProdOutMin=[]  UngainTsProdOutMax=[]  IntegratorContinuousStateAttributes=''  IntegratorStateMustResolveToSignalObject=off  IntegratorRTWStateStorageClass=Auto  FilterContinuousStateAttributes=''  FilterStateMustResolveToSignalObject=off  FilterRTWStateStorageClass=Auto  ParallelPVariant=InternalParameters  IdealPVariant=Disabled  IVariant=InternalParameters  DVariant=InternalParameters  IntegratorVariant=Continuous  SatVariant=Disabled  AWVariant=Passthrough  PCopyVariant=Disabled  TRVariant=Disabled  FdbkBlocksVariant=Forward  IdealPFdbkVariant=Disabled  SatFdbkVariant=Disabled  DerivativeFilterVariant=ContFilter  NVariant=InternalParameters  NCopyVariant=Disabled  FilterICVariant=InternalICsFilter  IntegratorICVariant=InternalICs  ExternalResetVariant=Disabled  TRSumVariant=Passthrough  SumFdbkVariant=Disabled  SumVariant=Sum_PID  TsampFilterVariant=InternalTs  TsampNgainVariant=Passthrough  TsampIntegralVariant=Passthrough  ExternalSaturationOutDataTypeStr=Inherit: Same as second input  aMode=0
  Ref_p1 : Constant  Value=[10;-10]  VectorParams1D=off
  Ref_v1 : Constant  Value=[0;0]  VectorParams1D=off
  Sum : Sum  Inputs=+-|
  Sum1 : Sum  Inputs=|-+
  u03 : Outport
  wires:
  x_rob2/1 -> Demux/1
  Demux/1 -> Sum/2
  Ref_p1/1 -> Sum/1
  Demux/2 -> Sum1/1
  Ref_v1/1 -> Sum1/2
  Add/1 -> u03/1
  Demux1/2 -> Add/2
  Demux1/1 -> Add/1
  Sum1/1 -> Mux/2
  Sum/1 -> Mux/1
  PID Controller/1 -> Demux1/1
  Mux/1 -> PID Controller/1

== system Experiment1_model/Controller1 PID/controller robot4 ==
  x_rob2 : Inport
  Add : Sum
  Demux : Demux  Outputs=2
  Demux1 : Demux  Outputs=2
  Mux : Mux  Inputs=2
  PID Controller : slpidlib/PID Controller  Controller=PID  Form=Parallel  TimeDomain=Continuous-time  UseExternalTs=off  SampleTime=-1  IntegratorMethod=Forward Euler  FilterMethod=Forward Euler  ControllerParametersSource=internal  P=5  I=0.0000001  UseKiTs=off  D=0.01  N=1  UseFilter=on  TunerSelectOption=Transfer Function Based (PID Tuner App)  InitialConditionSource=internal  InitialConditionForIntegrator=0  InitialConditionForFilter=0  DifferentiatorICPrevScaledInput=0  ExternalReset=none  TrackingMode=off  Kt=1  LimitOutput=off  SatLimitsSource=internal  UpperSaturationLimit=inf  LowerSaturationLimit=-inf  LinearizeAsGain=on  AntiWindupMode=none  Kb=1  POutMin=[]  POutMax=[]  IOutMin=[]  IOutMax=[]  DOutMin=[]  DOutMax=[]  NOutMin=[]  NOutMax=[]  SumOutMin=[]  SumOutMax=[]  SaturationOutMin=[]  SaturationOutMax=[]  PParamMin=[]  PParamMax=[]  IParamMin=[]  IParamMax=[]  DParamMin=[]  DParamMax=[]  NParamMin=[]  NParamMax=[]  KbParamMin=[]  KbParamMax=[]  KtParamMin=[]  KtParamMax=[]  KbOutMin=[]  KbOutMax=[]  KtOutMin=[]  KtOutMax=[]  IntegratorOutMin=[]  IntegratorOutMax=[]  FilterOutMin=[]  FilterOutMax=[]  SumI1OutMin=[]  SumI1OutMax=[]  SumI2OutMin=[]  SumI2OutMax=[]  SumI3OutMin=[]  SumI3OutMax=[]  SumI4OutMin=[]  SumI4OutMax=[]  SumDOutMin=[]  SumDOutMax=[]  DifferentiatorOutMin=[]  DifferentiatorOutMax=[]  FilterDiffOutCoefMin=[]  FilterDiffOutCoefMax=[]  ReciprocalOutMin=[]  ReciprocalOutMax=[]  SumDenOutMin=[]  SumDenOutMax=[]  SumNumOutMin=[]  SumNumOutMax=[]  DivideOutMin=[]  DivideOutMax=[]  UdiffTsProdOutMin=[]  UdiffTsProdOutMax=[]  NTsProdOutMin=[]  NTsProdOutMax=[]  UintegralTsProdOutMin=[]  UintegralTsProdOutMax=[]  UngainTsProdOutMin=[]  UngainTsProdOutMax=[]  IntegratorContinuousStateAttributes=''  IntegratorStateMustResolveToSignalObject=off  IntegratorRTWStateStorageClass=Auto  FilterContinuousStateAttributes=''  FilterStateMustResolveToSignalObject=off  FilterRTWStateStorageClass=Auto  ParallelPVariant=InternalParameters  IdealPVariant=Disabled  IVariant=InternalParameters  DVariant=InternalParameters  IntegratorVariant=Continuous  SatVariant=Disabled  AWVariant=Passthrough  PCopyVariant=Disabled  TRVariant=Disabled  FdbkBlocksVariant=Forward  IdealPFdbkVariant=Disabled  SatFdbkVariant=Disabled  DerivativeFilterVariant=ContFilter  NVariant=InternalParameters  NCopyVariant=Disabled  FilterICVariant=InternalICsFilter  IntegratorICVariant=InternalICs  ExternalResetVariant=Disabled  TRSumVariant=Passthrough  SumFdbkVariant=Disabled  SumVariant=Sum_PID  TsampFilterVariant=InternalTs  TsampNgainVariant=Passthrough  TsampIntegralVariant=Passthrough  ExternalSaturationOutDataTypeStr=Inherit: Same as second input  aMode=0
  Ref_p1 : Constant  Value=[0;-10]  VectorParams1D=off
  Ref_v1 : Constant  Value=[0;0]  VectorParams1D=off
  Sum : Sum  Inputs=+-|
  Sum1 : Sum  Inputs=|-+
  u04 : Outport
  wires:
  x_rob2/1 -> Demux/1
  Demux/1 -> Sum/2
  Ref_p1/1 -> Sum/1
  Demux/2 -> Sum1/1
  Ref_v1/1 -> Sum1/2
  PID Controller/1 -> Demux1/1
  Demux1/2 -> Add/2
  Add/1 -> u04/1
  Demux1/1 -> Add/1
  Mux/1 -> PID Controller/1
  Sum1/1 -> Mux/2
  Sum/1 -> Mux/1

== system Experiment1_model/Controller1 PID/controller robot5 ==
  x_rob2 : Inport
  Add : Sum
  Demux : Demux  Outputs=2
  Demux1 : Demux  Outputs=2
  Mux : Mux  Inputs=2
  PID Controller : slpidlib/PID Controller  Controller=PID  Form=Parallel  TimeDomain=Continuous-time  UseExternalTs=off  SampleTime=-1  IntegratorMethod=Forward Euler  FilterMethod=Forward Euler  ControllerParametersSource=internal  P=5  I=0  UseKiTs=off  D=0  N=100  UseFilter=on  TunerSelectOption=Transfer Function Based (PID Tuner App)  InitialConditionSource=internal  InitialConditionForIntegrator=0  InitialConditionForFilter=0  DifferentiatorICPrevScaledInput=0  ExternalReset=none  TrackingMode=off  Kt=1  LimitOutput=off  SatLimitsSource=internal  UpperSaturationLimit=inf  LowerSaturationLimit=-inf  LinearizeAsGain=on  AntiWindupMode=none  Kb=1  POutMin=[]  POutMax=[]  IOutMin=[]  IOutMax=[]  DOutMin=[]  DOutMax=[]  NOutMin=[]  NOutMax=[]  SumOutMin=[]  SumOutMax=[]  SaturationOutMin=[]  SaturationOutMax=[]  PParamMin=[]  PParamMax=[]  IParamMin=[]  IParamMax=[]  DParamMin=[]  DParamMax=[]  NParamMin=[]  NParamMax=[]  KbParamMin=[]  KbParamMax=[]  KtParamMin=[]  KtParamMax=[]  KbOutMin=[]  KbOutMax=[]  KtOutMin=[]  KtOutMax=[]  IntegratorOutMin=[]  IntegratorOutMax=[]  FilterOutMin=[]  FilterOutMax=[]  SumI1OutMin=[]  SumI1OutMax=[]  SumI2OutMin=[]  SumI2OutMax=[]  SumI3OutMin=[]  SumI3OutMax=[]  SumI4OutMin=[]  SumI4OutMax=[]  SumDOutMin=[]  SumDOutMax=[]  DifferentiatorOutMin=[]  DifferentiatorOutMax=[]  FilterDiffOutCoefMin=[]  FilterDiffOutCoefMax=[]  ReciprocalOutMin=[]  ReciprocalOutMax=[]  SumDenOutMin=[]  SumDenOutMax=[]  SumNumOutMin=[]  SumNumOutMax=[]  DivideOutMin=[]  DivideOutMax=[]  UdiffTsProdOutMin=[]  UdiffTsProdOutMax=[]  NTsProdOutMin=[]  NTsProdOutMax=[]  UintegralTsProdOutMin=[]  UintegralTsProdOutMax=[]  UngainTsProdOutMin=[]  UngainTsProdOutMax=[]  IntegratorContinuousStateAttributes=''  IntegratorStateMustResolveToSignalObject=off  IntegratorRTWStateStorageClass=Auto  FilterContinuousStateAttributes=''  FilterStateMustResolveToSignalObject=off  FilterRTWStateStorageClass=Auto  ParallelPVariant=InternalParameters  IdealPVariant=Disabled  IVariant=InternalParameters  DVariant=InternalParameters  IntegratorVariant=Continuous  SatVariant=Disabled  AWVariant=Passthrough  PCopyVariant=Disabled  TRVariant=Disabled  FdbkBlocksVariant=Forward  IdealPFdbkVariant=Disabled  SatFdbkVariant=Disabled  DerivativeFilterVariant=ContFilter  NVariant=InternalParameters  NCopyVariant=Disabled  FilterICVariant=InternalICsFilter  IntegratorICVariant=InternalICs  ExternalResetVariant=Disabled  TRSumVariant=Passthrough  SumFdbkVariant=Disabled  SumVariant=Sum_PID  TsampFilterVariant=InternalTs  TsampNgainVariant=Passthrough  TsampIntegralVariant=Passthrough  ExternalSaturationOutDataTypeStr=Inherit: Same as second input  aMode=0
  Ref_p1 : Constant  Value=[0;10]  VectorParams1D=off
  Ref_v1 : Constant  Value=[0;0]  VectorParams1D=off
  Sum : Sum  Inputs=+-|
  Sum1 : Sum  Inputs=|-+
  u05 : Outport
  wires:
  x_rob2/1 -> Demux/1
  Demux/1 -> Sum/2
  Ref_p1/1 -> Sum/1
  Demux/2 -> Sum1/1
  Ref_v1/1 -> Sum1/2
  Add/1 -> u05/1
  PID Controller/1 -> Demux1/1
  Demux1/2 -> Add/2
  Demux1/1 -> Add/1
  Mux/1 -> PID Controller/1
  Sum1/1 -> Mux/2
  Sum/1 -> Mux/1

== system Experiment1_model/Controller1 PID/controller robot6 ==
  x_rob2 : Inport
  Add : Sum
  Demux : Demux  Outputs=2
  Demux1 : Demux  Outputs=2
  Mux : Mux  Inputs=2
  PID Controller : slpidlib/PID Controller  Controller=PID  Form=Parallel  TimeDomain=Continuous-time  UseExternalTs=off  SampleTime=-1  IntegratorMethod=Forward Euler  FilterMethod=Forward Euler  ControllerParametersSource=internal  P=5  I=0  UseKiTs=off  D=0  N=100  UseFilter=on  TunerSelectOption=Transfer Function Based (PID Tuner App)  InitialConditionSource=internal  InitialConditionForIntegrator=0  InitialConditionForFilter=0  DifferentiatorICPrevScaledInput=0  ExternalReset=none  TrackingMode=off  Kt=1  LimitOutput=off  SatLimitsSource=internal  UpperSaturationLimit=inf  LowerSaturationLimit=-inf  LinearizeAsGain=on  AntiWindupMode=none  Kb=1  POutMin=[]  POutMax=[]  IOutMin=[]  IOutMax=[]  DOutMin=[]  DOutMax=[]  NOutMin=[]  NOutMax=[]  SumOutMin=[]  SumOutMax=[]  SaturationOutMin=[]  SaturationOutMax=[]  PParamMin=[]  PParamMax=[]  IParamMin=[]  IParamMax=[]  DParamMin=[]  DParamMax=[]  NParamMin=[]  NParamMax=[]  KbParamMin=[]  KbParamMax=[]  KtParamMin=[]  KtParamMax=[]  KbOutMin=[]  KbOutMax=[]  KtOutMin=[]  KtOutMax=[]  IntegratorOutMin=[]  IntegratorOutMax=[]  FilterOutMin=[]  FilterOutMax=[]  SumI1OutMin=[]  SumI1OutMax=[]  SumI2OutMin=[]  SumI2OutMax=[]  SumI3OutMin=[]  SumI3OutMax=[]  SumI4OutMin=[]  SumI4OutMax=[]  SumDOutMin=[]  SumDOutMax=[]  DifferentiatorOutMin=[]  DifferentiatorOutMax=[]  FilterDiffOutCoefMin=[]  FilterDiffOutCoefMax=[]  ReciprocalOutMin=[]  ReciprocalOutMax=[]  SumDenOutMin=[]  SumDenOutMax=[]  SumNumOutMin=[]  SumNumOutMax=[]  DivideOutMin=[]  DivideOutMax=[]  UdiffTsProdOutMin=[]  UdiffTsProdOutMax=[]  NTsProdOutMin=[]  NTsProdOutMax=[]  UintegralTsProdOutMin=[]  UintegralTsProdOutMax=[]  UngainTsProdOutMin=[]  UngainTsProdOutMax=[]  IntegratorContinuousStateAttributes=''  IntegratorStateMustResolveToSignalObject=off  IntegratorRTWStateStorageClass=Auto  FilterContinuousStateAttributes=''  FilterStateMustResolveToSignalObject=off  FilterRTWStateStorageClass=Auto  ParallelPVariant=InternalParameters  IdealPVariant=Disabled  IVariant=InternalParameters  DVariant=InternalParameters  IntegratorVariant=Continuous  SatVariant=Disabled  AWVariant=Passthrough  PCopyVariant=Disabled  TRVariant=Disabled  FdbkBlocksVariant=Forward  IdealPFdbkVariant=Disabled  SatFdbkVariant=Disabled  DerivativeFilterVariant=ContFilter  NVariant=InternalParameters  NCopyVariant=Disabled  FilterICVariant=InternalICsFilter  IntegratorICVariant=InternalICs  ExternalResetVariant=Disabled  TRSumVariant=Passthrough  SumFdbkVariant=Disabled  SumVariant=Sum_PID  TsampFilterVariant=InternalTs  TsampNgainVariant=Passthrough  TsampIntegralVariant=Passthrough  ExternalSaturationOutDataTypeStr=Inherit: Same as second input  aMode=0
  Ref_p1 : Constant  Value=[-12;-6]  VectorParams1D=off
  Ref_v1 : Constant  Value=[0;0]  VectorParams1D=off
  Sum : Sum  Inputs=+-|
  Sum1 : Sum  Inputs=|-+
  u06 : Outport
  wires:
  x_rob2/1 -> Demux/1
  Demux/1 -> Sum/2
  Ref_p1/1 -> Sum/1
  Demux/2 -> Sum1/1
  Ref_v1/1 -> Sum1/2
  PID Controller/1 -> Demux1/1
  Demux1/2 -> Add/2
  Add/1 -> u06/1
  Demux1/1 -> Add/1
  Mux/1 -> PID Controller/1
  Sum1/1 -> Mux/2
  Sum/1 -> Mux/1

== system Experiment1_model/Controller1 PID/controller robot7 ==
  x_rob2 : Inport
  Add : Sum
  Demux : Demux  Outputs=2
  Demux1 : Demux  Outputs=2
  Mux : Mux  Inputs=2
  PID Controller : slpidlib/PID Controller  Controller=PID  Form=Parallel  TimeDomain=Continuous-time  UseExternalTs=off  SampleTime=-1  IntegratorMethod=Forward Euler  FilterMethod=Forward Euler  ControllerParametersSource=internal  P=5  I=0  UseKiTs=off  D=0  N=100  UseFilter=on  TunerSelectOption=Transfer Function Based (PID Tuner App)  InitialConditionSource=internal  InitialConditionForIntegrator=0  InitialConditionForFilter=0  DifferentiatorICPrevScaledInput=0  ExternalReset=none  TrackingMode=off  Kt=1  LimitOutput=off  SatLimitsSource=internal  UpperSaturationLimit=inf  LowerSaturationLimit=-inf  LinearizeAsGain=on  AntiWindupMode=none  Kb=1  POutMin=[]  POutMax=[]  IOutMin=[]  IOutMax=[]  DOutMin=[]  DOutMax=[]  NOutMin=[]  NOutMax=[]  SumOutMin=[]  SumOutMax=[]  SaturationOutMin=[]  SaturationOutMax=[]  PParamMin=[]  PParamMax=[]  IParamMin=[]  IParamMax=[]  DParamMin=[]  DParamMax=[]  NParamMin=[]  NParamMax=[]  KbParamMin=[]  KbParamMax=[]  KtParamMin=[]  KtParamMax=[]  KbOutMin=[]  KbOutMax=[]  KtOutMin=[]  KtOutMax=[]  IntegratorOutMin=[]  IntegratorOutMax=[]  FilterOutMin=[]  FilterOutMax=[]  SumI1OutMin=[]  SumI1OutMax=[]  SumI2OutMin=[]  SumI2OutMax=[]  SumI3OutMin=[]  SumI3OutMax=[]  SumI4OutMin=[]  SumI4OutMax=[]  SumDOutMin=[]  SumDOutMax=[]  DifferentiatorOutMin=[]  DifferentiatorOutMax=[]  FilterDiffOutCoefMin=[]  FilterDiffOutCoefMax=[]  ReciprocalOutMin=[]  ReciprocalOutMax=[]  SumDenOutMin=[]  SumDenOutMax=[]  SumNumOutMin=[]  SumNumOutMax=[]  DivideOutMin=[]  DivideOutMax=[]  UdiffTsProdOutMin=[]  UdiffTsProdOutMax=[]  NTsProdOutMin=[]  NTsProdOutMax=[]  UintegralTsProdOutMin=[]  UintegralTsProdOutMax=[]  UngainTsProdOutMin=[]  UngainTsProdOutMax=[]  IntegratorContinuousStateAttributes=''  IntegratorStateMustResolveToSignalObject=off  IntegratorRTWStateStorageClass=Auto  FilterContinuousStateAttributes=''  FilterStateMustResolveToSignalObject=off  FilterRTWStateStorageClass=Auto  ParallelPVariant=InternalParameters  IdealPVariant=Disabled  IVariant=InternalParameters  DVariant=InternalParameters  IntegratorVariant=Continuous  SatVariant=Disabled  AWVariant=Passthrough  PCopyVariant=Disabled  TRVariant=Disabled  FdbkBlocksVariant=Forward  IdealPFdbkVariant=Disabled  SatFdbkVariant=Disabled  DerivativeFilterVariant=ContFilter  NVariant=InternalParameters  NCopyVariant=Disabled  FilterICVariant=InternalICsFilter  IntegratorICVariant=InternalICs  ExternalResetVariant=Disabled  TRSumVariant=Passthrough  SumFdbkVariant=Disabled  SumVariant=Sum_PID  TsampFilterVariant=InternalTs  TsampNgainVariant=Passthrough  TsampIntegralVariant=Passthrough  ExternalSaturationOutDataTypeStr=Inherit: Same as second input  aMode=0
  Ref_p1 : Constant  Value=[-10;10]  VectorParams1D=off
  Ref_v1 : Constant  Value=[0;0]  VectorParams1D=off
  Sum : Sum  Inputs=+-|
  Sum1 : Sum  Inputs=|-+
  u07 : Outport
  wires:
  x_rob2/1 -> Demux/1
  Demux/1 -> Sum/2
  Ref_p1/1 -> Sum/1
  Demux/2 -> Sum1/1
  Ref_v1/1 -> Sum1/2
  PID Controller/1 -> Demux1/1
  Demux1/2 -> Add/2
  Add/1 -> u07/1
  Demux1/1 -> Add/1
  Mux/1 -> PID Controller/1
  Sum1/1 -> Mux/2
  Sum/1 -> Mux/1
